simulink model "model2_sim"  (R2017b)
settings: Solver=ode45  StartTime=0.0  StopTime=30  MaxStep=0.001  RelTol=1e-6  EnableMultiTasking=on
values from neighbouring files (symbols this model uses):
  damp_spring = 1    [model2.m]
  DC_delay = 0.005    [model2.m]
  DC_max_force = 800    [model2.m]
  feet_delay = 0.1    [model2.m]
  k_cutoffspring = 20000    [model2.m]
  k_spring = 2500    [model2.m]
  linear_act_delay = 0.1    [model2.m]
  linear_act_max = 0.5    [model2.m]
  linear_act_speed = 0.05    [model2.m]
  m_bed = 8    [model2.m]
  m_payload = m_bed + m_patient    (= 48)    [model2.m]
  max_offset = 0.1    [model2.m]
  noise_rate = 0.1    [model2.m]
  noise_rate_limit = 10    [model2.m]
  noise_start_time = 3    [model2.m]
  patient_sit_pace = 50    [model2.m]
libraries: simulink x7, vrlib x6
settings Model: Creator=Perttu  LastModifiedBy=Omistaja
settings SolverCC: InitialStep=0.0005
settings OptimizationCC: LifeSpan=inf
settings DebuggingCC: SFUnexpectedBacktrackingDiag=warning  SFNoUnconditionalDefaultTransitionDiag=warning  SFExecutionAtInitializationDiag=none
settings CodeAppCC: StateflowObjectComments=on
settings GRTTargetCC: TargetLangStandard=C89/C90 (ANSI)  GeneratePreprocessorConditionals=Disable all
settings ConfigComp: CovMetricSettings=dw  CovHtmlReporting=on  CovSaveCumulativeToWorkspaceVar=on  CovSaveSingleToWorkspaceVar=on  CovExternalEMLEnable=off

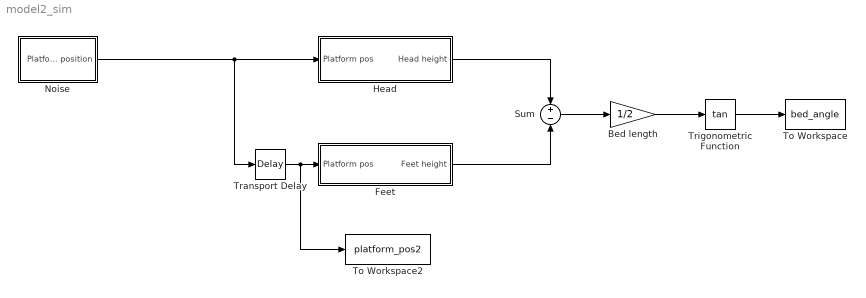
== system model2_sim ==
  Bed length : Gain  Gain=1/2
  Feet : Subsystem
  Head : Subsystem
  Noise : Subsystem
  Sum : Sum  Inputs=+|-
  To Workspace : ToWorkspace  VariableName=bed_angle  SaveFormat=Timeseries  SampleTime=-1
  To Workspace2 : ToWorkspace  VariableName=platform_pos2  SaveFormat=Timeseries  SampleTime=-1
  Transport Delay : TransportDelay  DelayTime=feet_delay
  Trigonometric Function : Trigonometry  Operator=tan
  wires:
  Feet/1(Feet height) -> Sum/2
  Head/1(Head height) -> Sum/1
  Sum/1 -> Bed length/1
  Bed length/1 -> Trigonometric Function/1
  Trigonometric Function/1 -> To Workspace/1
  Noise/1(Platform position) -> Transport Delay/1, Head/1(Platform pos)
  Transport Delay/1 -> To Workspace2/1, Feet/1(Platform pos)

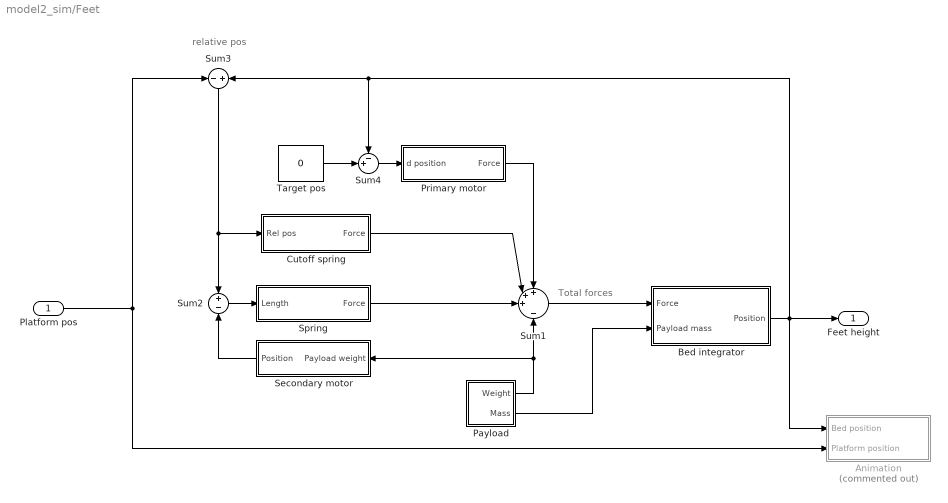
== system model2_sim/Feet ==
  note: Total forces
  note: relative pos
  Platform pos : Inport
  Animation : Subsystem  Commented=on
  Bed integrator : Subsystem
  Cutoff spring : Subsystem
  Payload : Subsystem
  Primary motor : Subsystem
  Secondary motor : Subsystem
  Spring : Subsystem
  Sum1 : Sum  Inputs=+++|-
  Sum2 : Sum  Inputs=+|-
  Sum3 : Sum  Inputs=-+
  Sum4 : Sum  Inputs=-+|
  Target pos : Constant  Value=0
  Feet height : Outport
  wires:
  Sum3/1 -> Cutoff spring/1(Rel pos), Sum2/1
  Cutoff spring/1(Force) -> Sum1/2
  Sum1/1 -> Bed integrator/1(Force)
  Payload/2(Mass) -> Bed integrator/2(Payload mass)
  Bed integrator/1(Position) -> Animation/1(Bed position), Feet height/1, Sum4/1, Sum3/2
  Spring/1(Force) -> Sum1/3
  Secondary motor/1(Position) -> Sum2/2
  Platform pos/1 -> Sum3/1, Animation/2(Platform position)
  Target pos/1 -> Sum4/2
  Sum4/1 -> Primary motor/1(d position)
  Payload/1(Weight) -> Secondary motor/1(Payload weight), Sum1/4
  Sum2/1 -> Spring/1(Length)
  Primary motor/1(Force) -> Sum1/1

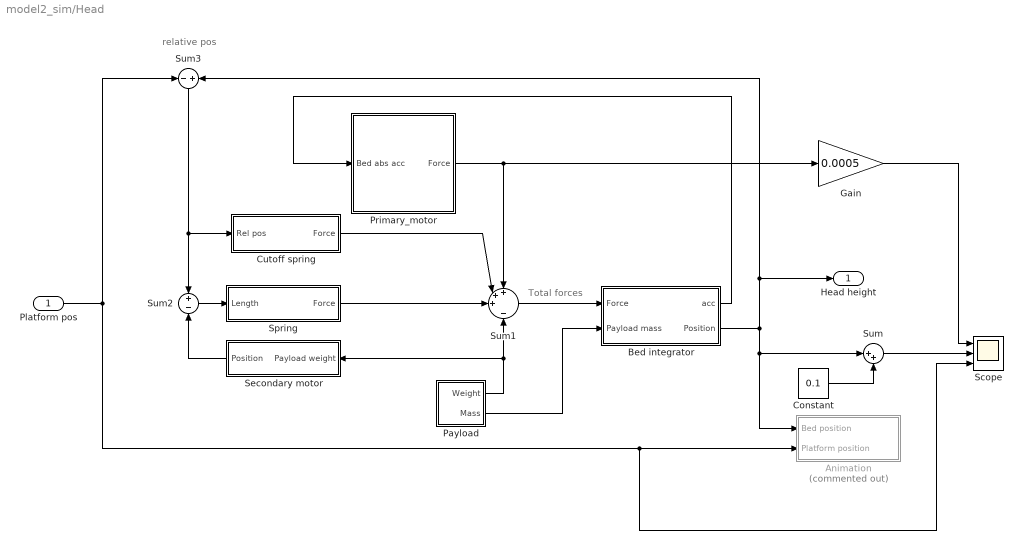
== system model2_sim/Head ==
  note: relative pos
  note: Total forces
  Platform pos : Inport
  Animation : Subsystem  Commented=on
  Bed integrator : Subsystem
  Constant : Constant  Value=0.1
  Cutoff spring : Subsystem
  Gain : Gain  Gain=0.0005
  Payload : Subsystem
  Primary_motor : Subsystem
  Scope : Scope  NumInputPorts=3
  Secondary motor : Subsystem
  Spring : Subsystem
  Sum : Sum  Inputs=|++
  Sum1 : Sum  Inputs=+++|-
  Sum2 : Sum  Inputs=+|-
  Sum3 : Sum  Inputs=-+
  Head height : Outport
  wires:
  Primary_motor/1(Force) -> Sum1/1, Gain/1
  Sum2/1 -> Spring/1(Length)
  Payload/1(Weight) -> Sum1/4, Secondary motor/1(Payload weight)
  Secondary motor/1(Position) -> Sum2/2
  Spring/1(Force) -> Sum1/3
  Bed integrator/2(Position) -> Sum3/2, Head height/1, Animation/1(Bed position), Sum/1
  Payload/2(Mass) -> Bed integrator/2(Payload mass)
  Sum1/1 -> Bed integrator/1(Force)
  Cutoff spring/1(Force) -> Sum1/2
  Sum3/1 -> Sum2/1, Cutoff spring/1(Rel pos)
  Bed integrator/1(acc) -> Primary_motor/1(Bed abs acc)
  Platform pos/1 -> Scope/3, Animation/2(Platform position), Sum3/1
  Constant/1 -> Sum/2
  Gain/1 -> Scope/1
  Sum/1 -> Scope/2

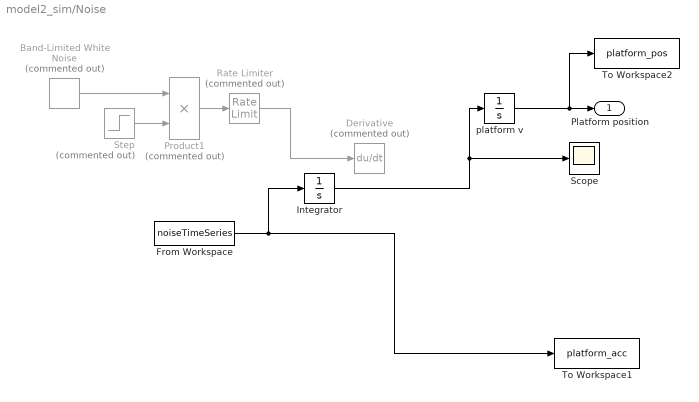
== system model2_sim/Noise ==
  Band-Limited White Noise : simulink/Sources/Band-Limited White Noise  Commented=on  Cov=noise_power  Ts=noise_rate  seed=noise_seed
  Derivative : Derivative  Commented=on
  From Workspace : FromWorkspace  VariableName=noiseTimeSeries  SampleTime=0
  Integrator : Integrator
  Product1 : Product  Commented=on  OutDataTypeStr=Inherit: Same as first input
  Rate Limiter : RateLimiter  Commented=on  RisingSlewLimit=noise_rate_limit  FallingSlewLimit=-noise_rate_limit
  Scope : Scope
  Step : Step  Commented=on  Time=noise_start_time  SampleTime=0
  To Workspace1 : ToWorkspace  VariableName=platform_acc  SaveFormat=Timeseries  SampleTime=-1
  To Workspace2 : ToWorkspace  VariableName=platform_pos  SaveFormat=Timeseries  SampleTime=-1
  platform v : Integrator
  Platform position : Outport
  wires:
  Band-Limited White Noise/1 -> Product1/1
  Step/1 -> Product1/2
  Product1/1 -> Rate Limiter/1
  platform v/1 -> To Workspace2/1, Platform position/1
  Rate Limiter/1 -> Derivative/1
  From Workspace/1 -> Integrator/1, To Workspace1/1
  Integrator/1 -> Scope/1, platform v/1

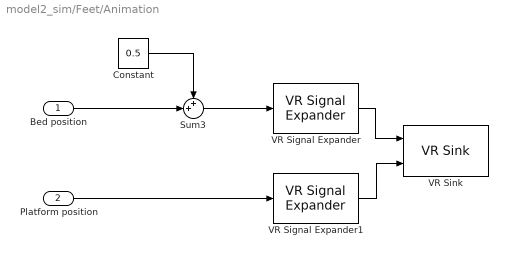
== system model2_sim/Feet/Animation ==
  Bed position : Inport
  Platform position : Inport  Port=2
  Constant : Constant  Value=0.5
  Sum3 : Sum  Inputs=++|
  VR Signal Expander : vrlib/VR Signal Expander  outwidth=3  outidx=[2]
      settings: SourceProductName=Simulink 3D Animation  SourceProductBaseCode=VR
  VR Signal Expander1 : vrlib/VR Signal Expander  outwidth=3  outidx=[2]
      settings: SourceProductName=Simulink 3D Animation  SourceProductBaseCode=VR
  VR Sink : vrlib/VR Sink  InstantiateOnLoad=on  SampleTime=0.03  ViewEnable=on  RemoteChange=off  RemoteView=off  FieldsWritten=Upper.translation.3.1.1.double#Lower.translation.3.1.1.double  WorldFileName=3dscene1.wrl  AutoView=off  VideoDimensions=[]  AllowVariableSize=off
      settings: SourceProductBaseCode=VR
  wires:
  Platform position/1 -> VR Signal Expander1/1
  Constant/1 -> Sum3/1
  Sum3/1 -> VR Signal Expander/1
  VR Signal Expander1/1 -> VR Sink/2
  VR Signal Expander/1 -> VR Sink/1
  Bed position/1 -> Sum3/2

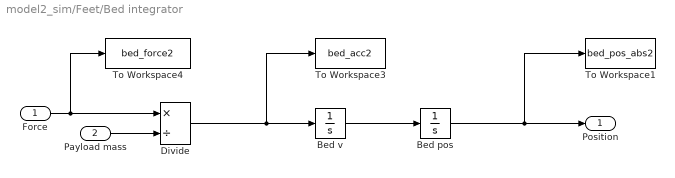
== system model2_sim/Feet/Bed integrator ==
  Force : Inport
  Payload mass : Inport  Port=2
  Bed pos : Integrator  UpperSaturationLimit=max_offset  LowerSaturationLimit=-max_offset  WrappedStateUpperValue=max_offset  WrappedStateLowerValue=-max_offset
  Bed v : Integrator
  Divide : Product  Inputs=*/
  To Workspace1 : ToWorkspace  VariableName=bed_pos_abs2  SaveFormat=Timeseries  SampleTime=-1
  To Workspace3 : ToWorkspace  VariableName=bed_acc2  SaveFormat=Timeseries  SampleTime=-1
  To Workspace4 : ToWorkspace  VariableName=bed_force2  SaveFormat=Timeseries  SampleTime=-1
  Position : Outport
  wires:
  Bed pos/1 -> Position/1, To Workspace1/1
  Payload mass/1 -> Divide/2
  Divide/1 -> Bed v/1, To Workspace3/1
  Bed v/1 -> Bed pos/1
  Force/1 -> To Workspace4/1, Divide/1

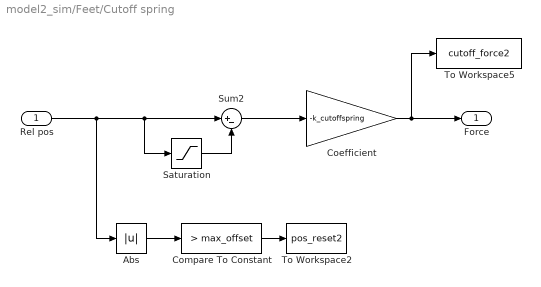
== system model2_sim/Feet/Cutoff spring ==
  Rel pos : Inport
  Abs : Abs
  Coefficient : Gain  Gain=-k_cutoffspring
  Compare To Constant : simulink/Logic and Bit Operations/Compare To Constant  relop=>  const=max_offset  OutDataTypeStr=boolean
  Saturation : Saturate  UpperLimit=max_offset  LowerLimit=-max_offset
  Sum2 : Sum  Inputs=|+-
  To Workspace2 : ToWorkspace  VariableName=pos_reset2  SaveFormat=Timeseries  SampleTime=-1
  To Workspace5 : ToWorkspace  VariableName=cutoff_force2  SaveFormat=Timeseries  SampleTime=-1
  Force : Outport
  wires:
  Coefficient/1 -> To Workspace5/1, Force/1
  Sum2/1 -> Coefficient/1
  Saturation/1 -> Sum2/2
  Abs/1 -> Compare To Constant/1
  Rel pos/1 -> Abs/1, Sum2/1, Saturation/1
  Compare To Constant/1 -> To Workspace2/1

== system model2_sim/Feet/Payload ==
  Payload weight : Gain  Gain=9.81
  Ramp : simulink/Sources/Ramp  slope=patient_sit_pace  start=patient_sit_time  X0=m_bed
  Saturation : Saturate  UpperLimit=m_payload  LowerLimit=0
  To Workspace5 : ToWorkspace  VariableName=payload_weight2  SaveFormat=Timeseries  SampleTime=-1
  Weight : Outport
  Mass : Outport  Port=2
  wires:
  Ramp/1 -> Saturation/1
  Saturation/1 -> Payload weight/1, Mass/1
  Payload weight/1 -> Weight/1, To Workspace5/1

== system model2_sim/Feet/Primary motor ==
  d position : Inport
  DC to workspace : ToWorkspace  VariableName=DC_force2  SaveFormat=Timeseries  SampleTime=-1
  PID Controller : simulink/Continuous/PID Controller  Controller=PID  TimeDomain=Continuous-time  SampleTime=-1  IntegratorMethod=Forward Euler  FilterMethod=Forward Euler  Form=Parallel  UseFilter=on  ControllerParametersSource=internal  P=0  I=0  D=0  N=1  InitialConditionSource=internal  InitialConditionForIntegrator=0  InitialConditionForFilter=0  ExternalReset=none  LimitOutput=off  UpperSaturationLimit=inf  LowerSaturationLimit=-inf  LinearizeAsGain=on  AntiWindupMode=none  Kb=1  TrackingMode=off  Kt=1  PParamMin=[]  PParamMax=[]  IParamMin=[]  IParamMax=[]  DParamMin=[]  DParamMax=[]  NParamMin=[]  NParamMax=[]  KbParamMin=[]  KbParamMax=[]  KtParamMin=[]  KtParamMax=[]  POutMin=[]  POutMax=[]  IOutMin=[]  IOutMax=[]  DOutMin=[]  DOutMax=[]  NOutMin=[]  NOutMax=[]  KbOutMin=[]  KbOutMax=[]  KtOutMin=[]  KtOutMax=[]  IntegratorOutMin=[]  IntegratorOutMax=[]  FilterOutMin=[]  FilterOutMax=[]  SumOutMin=[]  SumOutMax=[]  SumI1OutMin=[]  SumI1OutMax=[]  SumI2OutMin=[]  SumI2OutMax=[]  SumI3OutMin=[]  SumI3OutMax=[]  SumDOutMin=[]  SumDOutMax=[]  SaturationOutMin=[]  SaturationOutMax=[]  IntegratorContinuousStateAttributes=''  IntegratorStateMustResolveToSignalObject=off  IntegratorRTWStateStorageClass=Auto  FilterContinuousStateAttributes=''  FilterStateMustResolveToSignalObject=off  FilterRTWStateStorageClass=Auto  DifferentiatorICPrevScaledInput=0  DifferentiatorOutMin=[]  DifferentiatorOutMax=[]  InitialConditionSetting=State (most efficient)  FilterDiffOutCoefMin=[]  FilterDiffOutCoefMax=[]  SumDenOutMin=[]  SumDenOutMax=[]  SumNumOutMin=[]  SumNumOutMax=[]  ReciprocalOutMin=[]  ReciprocalOutMax=[]  DivideOutMin=[]  DivideOutMax=[]  TunerSelectOption=Transfer Function Based (PID Tuner App)
  Saturation : Saturate  UpperLimit=DC_max_force  LowerLimit=-DC_max_force
  Transport Delay : TransportDelay  DelayTime=DC_delay  BufferSize=4096
  Force : Outport
  wires:
  Transport Delay/1 -> PID Controller/1
  d position/1 -> Transport Delay/1
  PID Controller/1 -> Saturation/1
  Saturation/1 -> Force/1, DC to workspace/1

== system model2_sim/Feet/Secondary motor ==
  Payload weight : Inport
  Rate Limiter : RateLimiter  RisingSlewLimit=linear_act_speed  FallingSlewLimit=-linear_act_speed  SampleTimeMode=inherited  InitialCondition=m_bed * 9.81 / k_spring
  Saturation : Saturate  UpperLimit=linear_act_max  LowerLimit=0
  To Workspace6 : ToWorkspace  VariableName=lin_act_pos2  SaveFormat=Timeseries  SampleTime=-1
  Transport Delay : TransportDelay  DelayTime=linear_act_delay  InitialOutput=m_bed * 9.81 / k_spring  BufferSize=4096
  tgt pos : Gain  Gain=1/k_spring
  Position : Outport
  wires:
  tgt pos/1 -> Transport Delay/1
  Transport Delay/1 -> Rate Limiter/1
  Saturation/1 -> Position/1, To Workspace6/1
  Rate Limiter/1 -> Saturation/1
  Payload weight/1 -> tgt pos/1

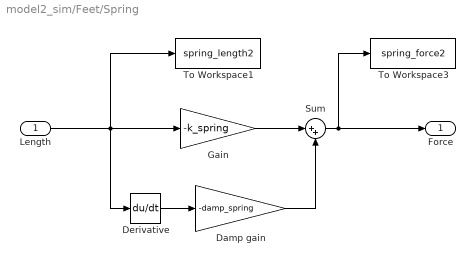
== system model2_sim/Feet/Spring ==
  Length : Inport
  Damp gain : Gain  Gain=-damp_spring
  Derivative : Derivative
  Gain : Gain  Gain=-k_spring
  Sum : Sum  Inputs=|++
  To Workspace1 : ToWorkspace  VariableName=spring_length2  SaveFormat=Timeseries  SampleTime=-1
  To Workspace3 : ToWorkspace  VariableName=spring_force2  SaveFormat=Timeseries  SampleTime=-1
  Force : Outport
  wires:
  Sum/1 -> Force/1, To Workspace3/1
  Damp gain/1 -> Sum/2
  Derivative/1 -> Damp gain/1
  Length/1 -> To Workspace1/1, Gain/1, Derivative/1
  Gain/1 -> Sum/1

== system model2_sim/Head/Animation ==
  Bed position : Inport
  Platform position : Inport  Port=2
  Constant : Constant  Value=0.5
  Sum3 : Sum  Inputs=++|
  VR Signal Expander : vrlib/VR Signal Expander  outwidth=3  outidx=[2]
      settings: SourceProductName=Simulink 3D Animation  SourceProductBaseCode=VR
  VR Signal Expander1 : vrlib/VR Signal Expander  outwidth=3  outidx=[2]
      settings: SourceProductName=Simulink 3D Animation  SourceProductBaseCode=VR
  VR Sink : vrlib/VR Sink  InstantiateOnLoad=on  SampleTime=0.03  ViewEnable=on  RemoteChange=off  RemoteView=off  FieldsWritten=Upper.translation.3.1.1.double#Lower.translation.3.1.1.double  WorldFileName=3dscene1.wrl  AutoView=off  VideoDimensions=[]  AllowVariableSize=off
      settings: SourceProductBaseCode=VR
  wires:
  Bed position/1 -> Sum3/2
  VR Signal Expander/1 -> VR Sink/1
  VR Signal Expander1/1 -> VR Sink/2
  Sum3/1 -> VR Signal Expander/1
  Constant/1 -> Sum3/1
  Platform position/1 -> VR Signal Expander1/1

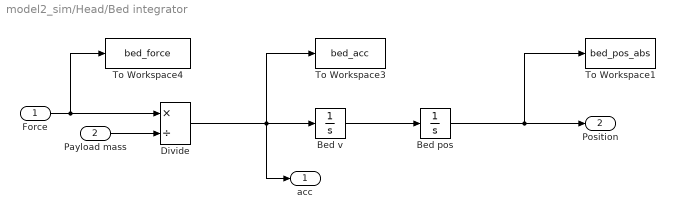
== system model2_sim/Head/Bed integrator ==
  Force : Inport
  Payload mass : Inport  Port=2
  Bed pos : Integrator  UpperSaturationLimit=max_offset  LowerSaturationLimit=-max_offset  WrappedStateUpperValue=max_offset  WrappedStateLowerValue=-max_offset
  Bed v : Integrator
  Divide : Product  Inputs=*/
  To Workspace1 : ToWorkspace  VariableName=bed_pos_abs  SaveFormat=Timeseries  SampleTime=-1
  To Workspace3 : ToWorkspace  VariableName=bed_acc  SaveFormat=Timeseries  SampleTime=-1
  To Workspace4 : ToWorkspace  VariableName=bed_force  SaveFormat=Timeseries  SampleTime=-1
  acc : Outport
  Position : Outport  Port=2
  wires:
  Force/1 -> Divide/1, To Workspace4/1
  Bed v/1 -> Bed pos/1
  Divide/1 -> acc/1, To Workspace3/1, Bed v/1
  Payload mass/1 -> Divide/2
  Bed pos/1 -> To Workspace1/1, Position/1

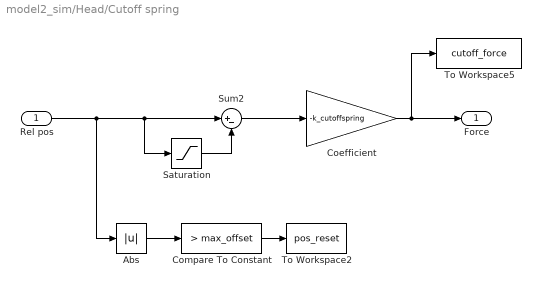
== system model2_sim/Head/Cutoff spring ==
  Rel pos : Inport
  Abs : Abs
  Coefficient : Gain  Gain=-k_cutoffspring
  Compare To Constant : simulink/Logic and Bit Operations/Compare To Constant  relop=>  const=max_offset  OutDataTypeStr=boolean
  Saturation : Saturate  UpperLimit=max_offset  LowerLimit=-max_offset
  Sum2 : Sum  Inputs=|+-
  To Workspace2 : ToWorkspace  VariableName=pos_reset  SaveFormat=Timeseries  SampleTime=-1
  To Workspace5 : ToWorkspace  VariableName=cutoff_force  SaveFormat=Timeseries  SampleTime=-1
  Force : Outport
  wires:
  Compare To Constant/1 -> To Workspace2/1
  Rel pos/1 -> Saturation/1, Sum2/1, Abs/1
  Abs/1 -> Compare To Constant/1
  Saturation/1 -> Sum2/2
  Sum2/1 -> Coefficient/1
  Coefficient/1 -> Force/1, To Workspace5/1

== system model2_sim/Head/Payload ==
  Payload weight : Gain  Gain=9.81
  Ramp : simulink/Sources/Ramp  slope=patient_sit_pace  start=patient_sit_time  X0=m_bed
  Saturation : Saturate  UpperLimit=m_payload  LowerLimit=0
  To Workspace5 : ToWorkspace  VariableName=payload_weight  SaveFormat=Timeseries  SampleTime=-1
  Weight : Outport
  Mass : Outport  Port=2
  wires:
  Payload weight/1 -> To Workspace5/1, Weight/1
  Saturation/1 -> Mass/1, Payload weight/1
  Ramp/1 -> Saturation/1

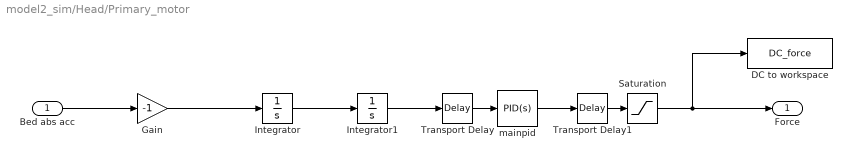
== system model2_sim/Head/Primary_motor ==
  Bed abs acc : Inport
  DC to workspace : ToWorkspace  VariableName=DC_force  SaveFormat=Timeseries  SampleTime=-1
  Gain : Gain  Gain=-1
  Integrator : Integrator
  Integrator1 : Integrator
  Saturation : Saturate  UpperLimit=DC_max_force  LowerLimit=-DC_max_force
  Transport Delay : TransportDelay  DelayTime=DC_delay  BufferSize=4096
  Transport Delay1 : TransportDelay  DelayTime=0.001  BufferSize=4096
  mainpid : simulink/Continuous/PID Controller  Controller=PID  TimeDomain=Continuous-time  SampleTime=-1  IntegratorMethod=Forward Euler  FilterMethod=Forward Euler  Form=Parallel  UseFilter=on  ControllerParametersSource=internal  P=0  I=0  D=840  N=104  InitialConditionSource=internal  InitialConditionForIntegrator=0  InitialConditionForFilter=0  ExternalReset=none  LimitOutput=off  UpperSaturationLimit=inf  LowerSaturationLimit=-inf  LinearizeAsGain=on  AntiWindupMode=none  Kb=1  TrackingMode=off  Kt=1  PParamMin=[]  PParamMax=[]  IParamMin=[]  IParamMax=[]  DParamMin=[]  DParamMax=[]  NParamMin=[]  NParamMax=[]  KbParamMin=[]  KbParamMax=[]  KtParamMin=[]  KtParamMax=[]  POutMin=[]  POutMax=[]  IOutMin=[]  IOutMax=[]  DOutMin=[]  DOutMax=[]  NOutMin=[]  NOutMax=[]  KbOutMin=[]  KbOutMax=[]  KtOutMin=[]  KtOutMax=[]  IntegratorOutMin=[]  IntegratorOutMax=[]  FilterOutMin=[]  FilterOutMax=[]  SumOutMin=[]  SumOutMax=[]  SumI1OutMin=[]  SumI1OutMax=[]  SumI2OutMin=[]  SumI2OutMax=[]  SumI3OutMin=[]  SumI3OutMax=[]  SumDOutMin=[]  SumDOutMax=[]  SaturationOutMin=[]  SaturationOutMax=[]  IntegratorContinuousStateAttributes=''  IntegratorStateMustResolveToSignalObject=off  IntegratorRTWStateStorageClass=Auto  FilterContinuousStateAttributes=''  FilterStateMustResolveToSignalObject=off  FilterRTWStateStorageClass=Auto  DifferentiatorICPrevScaledInput=0  DifferentiatorOutMin=[]  DifferentiatorOutMax=[]  InitialConditionSetting=State (most efficient)  FilterDiffOutCoefMin=[]  FilterDiffOutCoefMax=[]  SumDenOutMin=[]  SumDenOutMax=[]  SumNumOutMin=[]  SumNumOutMax=[]  ReciprocalOutMin=[]  ReciprocalOutMax=[]  DivideOutMin=[]  DivideOutMax=[]  TunerSelectOption=Transfer Function Based (PID Tuner App)
  Force : Outport
  wires:
  Transport Delay/1 -> mainpid/1
  Transport Delay1/1 -> Saturation/1
  mainpid/1 -> Transport Delay1/1
  Saturation/1 -> Force/1, DC to workspace/1
  Integrator/1 -> Integrator1/1
  Integrator1/1 -> Transport Delay/1
  Bed abs acc/1 -> Gain/1
  Gain/1 -> Integrator/1

== system model2_sim/Head/Secondary motor ==
  Payload weight : Inport
  Rate Limiter : RateLimiter  RisingSlewLimit=linear_act_speed  FallingSlewLimit=-linear_act_speed  SampleTimeMode=inherited  InitialCondition=m_bed * 9.81 / k_spring
  Saturation : Saturate  UpperLimit=linear_act_max  LowerLimit=0
  To Workspace6 : ToWorkspace  VariableName=lin_act_pos  SaveFormat=Timeseries  SampleTime=-1
  Transport Delay : TransportDelay  DelayTime=linear_act_delay  InitialOutput=m_bed * 9.81 / k_spring  BufferSize=4096
  tgt pos : Gain  Gain=1/k_spring
  Position : Outport
  wires:
  Payload weight/1 -> tgt pos/1
  Rate Limiter/1 -> Saturation/1
  Saturation/1 -> To Workspace6/1, Position/1
  Transport Delay/1 -> Rate Limiter/1
  tgt pos/1 -> Transport Delay/1

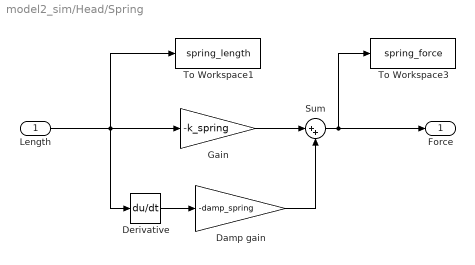
== system model2_sim/Head/Spring ==
  Length : Inport
  Damp gain : Gain  Gain=-damp_spring
  Derivative : Derivative
  Gain : Gain  Gain=-k_spring
  Sum : Sum  Inputs=|++
  To Workspace1 : ToWorkspace  VariableName=spring_length  SaveFormat=Timeseries  SampleTime=-1
  To Workspace3 : ToWorkspace  VariableName=spring_force  SaveFormat=Timeseries  SampleTime=-1
  Force : Outport
  wires:
  Gain/1 -> Sum/1
  Length/1 -> Derivative/1, Gain/1, To Workspace1/1
  Derivative/1 -> Damp gain/1
  Damp gain/1 -> Sum/2
  Sum/1 -> To Workspace3/1, Force/1
